simulink model "atrias_boom_nmSt_kinSw_v4"  (R2015a)
settings: Solver=ode23t  StartTime=0.0  StopTime=t_end  FixedStep=0.001  MaxStep=1e-3  RelTol=1e-3
InitFcn:
  | addpath('../common/')
  | colors
StartFcn:
  | tic
StopFcn:
  | %stopscript
values from neighbouring files (symbols this model uses):
  dt_a_dTrunk_boom = 5    [main_1_nmSt_kinSw.m]    (also in main_2_nmSt_kinSw_v2.m; main_3_nmSt_kinSw_v3.m; main_4_nmSt_kinSw_v4.m)
  dt_fade_boomCtrl = 2    [main_1_nmSt_kinSw.m]    (also in main_2_nmSt_kinSw_v2.m; main_3_nmSt_kinSw_v3.m; main_4_nmSt_kinSw_v4.m)
  initial_boom_yaw = 15*pi/180    (= 0.261799387799)    [main_2_nmSt_kinSw_v2.m]    (also in main_3_nmSt_kinSw_v3.m; main_4_nmSt_kinSw_v4.m)
  kd_boom_roll_Ctrl = 0    [main_1_nmSt_kinSw - Copy.m]    (also in main_1_nmSt_kinSw.m; main_2_nmSt_kinSw_v2.m; main_3_nmSt_kinSw_v3.m; main_4_nmSt_kinSw_v4.m)
  kd_boom_yaw_Ctrl = 0.1*kp_boom_yaw_Ctrl    (= 100000000)    [main_1_nmSt_kinSw - Copy.m]    (also in main_1_nmSt_kinSw.m = 1000000000; main_2_nmSt_kinSw_v2.m = 10000000; main_3_nmSt_kinSw_v3.m = 10000000; main_4_nmSt_kinSw_v4.m = 10000000)
  kd_motor = 0.90*2*sqrt(3.75*kp_motor)    [main_1_nmSt_kinSw - Copy.m]
  kinSw_alpha_start = 100*pi/180    (= 1.74532925199)    [main_1_nmSt_kinSw - Copy.m]    (also in main_1_nmSt_kinSw.m = 1.91986217719; main_2_nmSt_kinSw_v2.m = 1.83259571459; main_3_nmSt_kinSw_v3.m = 1.83259571459; main_4_nmSt_kinSw_v4.m = 1.83259571459)
  kinSw_alpha_tgt = 80*pi/180    (= 1.3962634016)    [main_1_nmSt_kinSw - Copy.m]    (also in main_1_nmSt_kinSw.m = 1.2217304764; main_2_nmSt_kinSw_v2.m = 1.2217304764; main_3_nmSt_kinSw_v3.m = 1.2217304764; main_4_nmSt_kinSw_v4.m = 1.2217304764)
  kinSw_t_start = 1.5    [main_1_nmSt_kinSw - Copy.m]    (also in main_1_nmSt_kinSw.m; main_2_nmSt_kinSw_v2.m = 0.5; main_3_nmSt_kinSw_v3.m = 0.5; main_4_nmSt_kinSw_v4.m = 0.5)
  kp_boom_roll_Ctrl = 0    [main_1_nmSt_kinSw - Copy.m]    (also in main_1_nmSt_kinSw.m; main_2_nmSt_kinSw_v2.m; main_3_nmSt_kinSw_v3.m; main_4_nmSt_kinSw_v4.m)
  kp_boom_yaw_Ctrl = 1e9    (= 1000000000)    [main_1_nmSt_kinSw - Copy.m]    (also in main_1_nmSt_kinSw.m = 10000000000; main_2_nmSt_kinSw_v2.m = 100000000; main_3_nmSt_kinSw_v3.m = 100000000; main_4_nmSt_kinSw_v4.m = 100000000)
  kp_motor = 3000    [main_1_nmSt_kinSw - Copy.m]
  max_back_bar_angle = 262.4*pi/180    (= 4.57974395723)    [main_1_nmSt_kinSw - Copy.m]
  max_front_bar_angle = 194.8*pi/180    (= 3.39990138288)    [main_1_nmSt_kinSw - Copy.m]
  min_back_bar_angle = 165.0*pi/180    (= 2.87979326579)    [main_1_nmSt_kinSw - Copy.m]
  min_front_bar_angle = 98.0*pi/180    (= 1.71042266695)    [main_1_nmSt_kinSw - Copy.m]
  poser_LLegAlp = (initial_l_leg_angle -pi/2)*180/pi    (= 105)    [main_2_nmSt_kinSw_v2.m]    (also in main_3_nmSt_kinSw_v3.m; main_4_nmSt_kinSw_v4.m)
  poser_LLegLen = initial_l_leg_length    (= 0.88)    [main_2_nmSt_kinSw_v2.m]    (also in main_3_nmSt_kinSw_v3.m; main_4_nmSt_kinSw_v4.m)
  poser_RLegAlp = (initial_r_leg_angle -pi/2)*180/pi    (= 75)    [main_2_nmSt_kinSw_v2.m]    (also in main_3_nmSt_kinSw_v3.m; main_4_nmSt_kinSw_v4.m)
  poser_RLegLen = initial_r_leg_length    (= 0.9)    [main_2_nmSt_kinSw_v2.m]    (also in main_3_nmSt_kinSw_v3.m; main_4_nmSt_kinSw_v4.m)
  tEnd_boomCtrl = t_end    (= 20)    [main_1_nmSt_kinSw - Copy.m]    (also in main_1_nmSt_kinSw.m = 3; main_2_nmSt_kinSw_v2.m = 7.5; main_3_nmSt_kinSw_v3.m = 7.5; main_4_nmSt_kinSw_v4.m = 7.5)
  tStart_boomCtrl = 1    [main_1_nmSt_kinSw - Copy.m]    (also in main_1_nmSt_kinSw.m = 0; main_2_nmSt_kinSw_v2.m = 0.5; main_3_nmSt_kinSw_v3.m = 0.5; main_4_nmSt_kinSw_v4.m = 0.5)
  tune_kinSw_alpha_start = kinSw_alpha_start*180/pi    (= 105)    [main_2_nmSt_kinSw_v2.m]    (also in main_3_nmSt_kinSw_v3.m; main_4_nmSt_kinSw_v4.m)
  tune_kinSw_alpha_tgt = kinSw_alpha_tgt*180/pi    (= 70)    [main_2_nmSt_kinSw_v2.m]    (also in main_3_nmSt_kinSw_v3.m; main_4_nmSt_kinSw_v4.m)
  tune_kinSw_gClr_tgt = kinSw_gClr    (= 0.15)    [main_4_nmSt_kinSw_v4.m]
  tune_kinSw_gH_tgt = kinSw_gH_tgt    (= -0.01)    [main_4_nmSt_kinSw_v4.m]
  tune_M1_G = St_FGain_VAS*FmaxVAS    [main_2_nmSt_kinSw_v2.m]    (also in main_3_nmSt_kinSw_v3.m; main_4_nmSt_kinSw_v4.m)
  tune_M3_0 = CtrlPar_theta0*180/pi    [main_2_nmSt_kinSw_v2.m]    (also in main_3_nmSt_kinSw_v3.m; main_4_nmSt_kinSw_v4.m)
  tune_M3_D = St_GainDTh_HFL    [main_2_nmSt_kinSw_v2.m]    (also in main_3_nmSt_kinSw_v3.m; main_4_nmSt_kinSw_v4.m)
  tune_M3_P = St_GainTh_HFL    [main_2_nmSt_kinSw_v2.m]    (also in main_3_nmSt_kinSw_v3.m; main_4_nmSt_kinSw_v4.m)
  tune_M4_G = 1    [main_3_nmSt_kinSw_v3.m]    (also in main_4_nmSt_kinSw_v4.m)
  v_dTrunk_boom = 1.3    [main_1_nmSt_kinSw.m]    (also in main_2_nmSt_kinSw_v2.m; main_3_nmSt_kinSw_v3.m; main_4_nmSt_kinSw_v4.m)
undefined symbols (not defined in the file or in its folder): A1_notch_f1, A2_notch_f1, A_lpf_dtau, A_lpf_velocity, ankle_stiffness, B1_lpf_dtau, B1_lpf_velocity, B1_notch_f1, B2_lpf_dtau, B2_lpf_velocity, B2_notch_f1, b_hmotor, b_leg_spring, b_rotor, base_color_d, boom_color_d, boom_mount_to_center_diagonal, breakaway_friction, c_jointstop, contactThr, coulomb_friction, d_com, delta_phi_max, delta_phi_max_buffer, delta_phi_max_dropoff, delta_phi_min, fblink_color_d, floor_color_d, FmaxBFSH, FmaxGLU, FmaxHAM, FmaxHFL, FmaxRF, FmaxVAS, foot_color_d, FPCtrlPar, friction_linear_zone, g, gain_nodes_sea_torque, HIP_MTR_MAX_CONT_TORQUE, HIP_MTR_MAX_TORQUE, hshaft_color_d, initial_boom_pitch, initial_boom_roll, initial_hip_roll, initial_winch_angle, j_motor, k_gn, k_gt, k_leg_spring, K_notch_f1, k_phi, k_sea, Kb_leg, kd_lateral, kd_shin_max, kd_shin_min, kd_splay_max, kd_splay_min, kd_thigh_max ... (+186)
libraries: sm_lib x210, nesl_utility x140, simulink x65, simulink_extras x32, fl_lib x16, mblibv1 x2, commnoisgen2 x1
(part 17 of 17)

== system atrias_boom_nmSt_kinSw_v4/Control/Behavior Control/Virtual Neuromuscular Control/Torque Distribution/mech limit avoidance1/PD Joint Limit1/R scale desired torque1 ==
  note: NOTE: min_splay_angle does not equal delta_phi_min
  phi_thigh [rad] : Inport
  phi_shin [rad] : Inport  Port=2
  k : Inport  Port=3
  Constant : Constant
  Constant1 : Constant  Value=delta_phi_max - delta_phi_max_buffer
  Constant10 : Constant  Value=phi_thigh_max_buffer
  Constant11 : Constant  Value=phi_shin_min_buffer
  Constant12 : Constant  Value=phi_shin_max_buffer
  Constant13 : Constant
  Constant2 : Constant  Value=phi_thigh_max - phi_thigh_max_buffer
  Constant3 : Constant  Value=min_splay_angle
  Constant4 : Constant  Value=phi_thigh_min + phi_thigh_min_buffer
  Constant5 : Constant  Value=phi_shin_max - phi_shin_max_buffer
  Constant6 : Constant  Value=phi_shin_min + phi_shin_min_buffer
  Constant7 : Constant  Value=min_splay_angle - delta_phi_min
  Constant8 : Constant  Value=delta_phi_max_buffer
  Constant9 : Constant  Value=phi_thigh_min_buffer
  Demux : Demux  Outputs=2
  Divide{,1..5} (6 alike) : Product  Inputs=/*
  Gain : Gain  Gain=-1
  Gain1 : Gain  Gain=-1
  Gain2 : Gain  Gain=-1
  L scale hip/knee : Scope  NumInputPorts=4
      settings: ShowLegends=on  TimeRange=2.5  YMin=-100~-5e+07~-1e+07~-5  YMax=100~1e+07~5e+07~5  SaveName=ScopeData5
  Mux{,3,7..8} (4 alike) : Mux  Inputs=2
  Sum : Sum  Inputs=|+-
  Sum1 : Sum  Inputs=-+|
  Sum2 : Sum  Inputs=+-
  Sum{3..8} (6 alike) : Sum  Inputs=+-|
  [0,1]{,1..6} (7 alike) : Saturate  UpperLimit=1  LowerLimit=0
  max : MinMax  Function=max  Inputs=4
  max1 : MinMax  Function=max  Inputs=4
  to hip_knee : MATLAB Function  TreatAsAtomicUnit=on
  scale_hip : Outport
  scale_knee : Outport  Port=2
  wires:
  "[0,1]6"/1 -> Demux/1
  Mux3/1 -> L scale hip/knee/4
  Demux/2 -> Sum1/1
  Demux/1 -> Sum/2
  to hip_knee/1(scale_hip_knee) -> "[0,1]6"/1
  k/1 -> to hip_knee/3(k)
  max1/1 -> to hip_knee/2(scale_front)
  max/1 -> to hip_knee/1(scale_back)
  Sum1/1 -> scale_knee/1, Mux3/2
  [min_thigh_scale] -> max1/3
  [max_thigh_scale] -> max1/4
  [max_splay_scale] -> max/4, max1/2
  [min_splay_scale] -> max/3, max1/1
  [max_shin_scale] -> max/2
  [min_shin_scale] -> max/1
  Constant13/1 -> Sum1/2
  Gain2/1 -> Divide5/2
  Constant12/1 -> Divide5/1
  Sum7/1 -> Gain2/1
  "[0,1]5"/1 -> [max_shin_scale]
  Divide5/1 -> "[0,1]5"/1
  Constant11/1 -> Divide4/1
  Sum8/1 -> Divide4/2
  "[0,1]4"/1 -> [min_shin_scale]
  Divide4/1 -> "[0,1]4"/1
  Constant10/1 -> Divide3/1
  Sum5/1 -> Gain1/1
  Gain1/1 -> Divide3/2
  "[0,1]3"/1 -> [max_thigh_scale]
  Divide3/1 -> "[0,1]3"/1
  Constant9/1 -> Divide2/1
  Sum6/1 -> Divide2/2
  "[0,1]2"/1 -> [min_thigh_scale]
  Divide2/1 -> "[0,1]2"/1
  Gain/1 -> Divide1/2
  Constant8/1 -> Divide1/1
  Sum3/1 -> Gain/1
  "[0,1]1"/1 -> [max_splay_scale]
  Divide1/1 -> "[0,1]1"/1
  "[0,1]"/1 -> [min_splay_scale]
  Divide/1 -> "[0,1]"/1
  Sum4/1 -> Divide/2
  Constant7/1 -> Divide/1
  Constant/1 -> Sum/1
  Sum/1 -> scale_hip/1, Mux3/1
  [max_splay_scale] -> Mux7/2  "max_splay_trq"
  [min_splay_scale] -> Mux7/1  "min_splay_trq"
  Mux7/1 -> L scale hip/knee/3
  Mux8/1 -> L scale hip/knee/2
  [max_shin_scale] -> Mux8/2  "max_shin_trq"
  [min_shin_scale] -> Mux8/1  "min_shin_trq"
  Mux/1 -> L scale hip/knee/1
  [max_thigh_scale] -> Mux/2  "max_thigh_trq"
  [min_thigh_scale] -> Mux/1  "min_thigh_trq"
  Constant5/1 -> Sum7/1
  [shin] -> Sum7/2
  Constant6/1 -> Sum8/1
  [shin] -> Sum8/2
  Constant2/1 -> Sum5/1
  [thigh] -> Sum5/2
  Constant4/1 -> Sum6/1
  [thigh] -> Sum6/2
  Constant1/1 -> Sum3/1
  [splay] -> Sum3/2
  Constant3/1 -> Sum4/1
  [splay] -> Sum4/2
  Sum2/1 -> [splay]  "splay angle"
  phi_thigh [rad]/1 -> Sum2/2, [thigh]
  phi_shin [rad]/1 -> Sum2/1, [shin]

== matlab function atrias_boom_nmSt_kinSw_v4/Control/Behavior Control/Virtual Neuromuscular Control/Torque Distribution/mech limit avoidance1/PD Joint Limit1/R scale desired torque/to hip_knee ==
  data: scale_back input; scale_hip_knee output; scale_front input; k input
function scale_hip_knee = fcn(scale_back,scale_front,k)

J_inv_trans = [1,1;
               -((k+1)/(2*k)),-((k-1)/(2*k))];
           
scale_hip_knee = J_inv_trans*[scale_back;scale_front];

== matlab function atrias_boom_nmSt_kinSw_v4/Control/Behavior Control/Virtual Neuromuscular Control/Torque Distribution/map_tau_R ==
  settings: updateMethod=DISCRETE  sampleTime=sample_time
  data: tauH_des input; tauB output; tauK_des input; tauF output; k input; Jinv_trans output
function [tauB,tauF, Jinv_trans] = map_virtual_torques(tauH_des,tauK_des,k)
%% FOR REFERENCE: 
%   [dphi_hip; dphi_knee] = J * [dq_back; dq_front];
%   
%   [dq_back; dq_front] = J^(-1) * [dphi_hip; dphi_knee];
%
%   [tauB; tauF] = Jt * [tauH, tauK]
%   
%   [tauH, tauK] = Jt^(-1) * [tauB; tauF]
%
%   J = [(1-k)/2    (1+k)/2 ]   where   k = l_s*sin((q_back-q_front)/2) /
%       [-k         k       ]               l_v*cos(phi_knee/2)
%
% 

%% Construct jacobian, then map virtual torques to actuator torques
j11 = (1-k)/2;
j12 = (1+k)/2;
j21 = -k;
j22 = k;

J = [j11, j12; j21, j22]; 
Jinv_trans = inv(J)';

tau_q = J'*[tauH_des; tauK_des];

tauB = tau_q(1);
tauF = tau_q(2);

end

== matlab function atrias_boom_nmSt_kinSw_v4/Control/Behavior Control/Virtual Neuromuscular Control/Torque Distribution/mech limit avoidance1/PD Joint Limit1/R scale desired torque1/to hip_knee ==
  data: scale_back input; scale_hip_knee output; scale_front input; k input
function scale_hip_knee = fcn(scale_back,scale_front,k)

J_inv_trans = [1,1;
               -((k+1)/(2*k)),-((k-1)/(2*k))];
           
scale_hip_knee = J_inv_trans*[scale_back;scale_front];

== matlab function atrias_boom_nmSt_kinSw_v4/Control/Behavior Control/Virtual Neuromuscular Control/Torque Distribution/map_tau_L ==
  settings: updateMethod=DISCRETE  sampleTime=sample_time
  data: tauH_des input; tauB output; tauK_des input; tauF output; k input; Jinv_trans output
function [tauB,tauF, Jinv_trans] = map_virtual_torques(tauH_des,tauK_des,k)
%% FOR REFERENCE: 
%   [dphi_hip; dphi_knee] = J * [dq_back; dq_front];
%   
%   [dq_back; dq_front] = J^(-1) * [dphi_hip; dphi_knee];
%
%   [tauB; tauF] = Jt * [tauH, tauK]
%   
%   [tauH, tauK] = Jt^(-1) * [tauB; tauF]
%
%   J = [(1-k)/2    (1+k)/2 ]   where   k = l_s*sin((q_back-q_front)/2) /
%       [-k         k       ]               l_v*cos(phi_knee/2)
%
% 

%% Construct jacobian, then map virtual torques to actuator torques
j11 = (1-k)/2;
j12 = (1+k)/2;
j21 = -k;
j22 = k;

J = [j11, j12; j21, j22]; 
Jinv_trans = inv(J)';

tau_q = J'*[tauH_des; tauK_des];

tauB = tau_q(1);
tauF = tau_q(2);

end

== matlab function atrias_boom_nmSt_kinSw_v4/Control/Behavior Control/Virtual Neuromuscular Control/Torque Distribution/mech limit avoidance1/PD Joint Limit1/to hip_knee ==
  data: Rtau_back input; tau_pd_hip_knee output; Rtau_front input; Ltau_back input; Ltau_front input; kR input; kL input
function tau_pd_hip_knee = fcn(Rtau_back,Rtau_front,Ltau_back,Ltau_front,kR,kL)

J_inv_trans = [1,1,0,0;
               -((kR+1)/(2*kR)),-((kR-1)/(2*kR)),0,0;
               0,0,1,1;
               0,0,-((kL+1)/(2*kL)),-((kL-1)/(2*kL))];
           
tau_pd_hip_knee = J_inv_trans*[Rtau_back;
                               Rtau_front;
                               Ltau_back;
                               Ltau_front];

== matlab function atrias_boom_nmSt_kinSw_v4/Control/Behavior Control/Lateral Motor Control/Lateral Control1 ==
  data: tau_r output size=1; qLateralR input; dqLateralR input; qLateralL input; dqLateralL input; F_leg_R input; F_leg_L input; lateral_transition_force parameter; lateral_target_angle_right parameter; m_leg_motor parameter; m_leg parameter; g parameter; lateral_offset parameter; tau_l output size=1; kp_lateral parameter; kd_lateral parameter; minimum_lateral_angle parameter; maximum_lateral_angle parameter; HIP_MTR_MAX_CONT_TORQUE parameter
function [tau_r, tau_l] = LateralBoomControl(...
    qLateralR, dqLateralR, qLateralL, dqLateralL, F_leg_R, F_leg_L,...
    lateral_transition_force, lateral_target_angle_right,...
    m_leg_motor, m_leg, g, lateral_offset,...
    kp_lateral, kd_lateral, minimum_lateral_angle, maximum_lateral_angle, HIP_MTR_MAX_CONT_TORQUE)
    
    % Only add gravity compensation to PD when suspended from winch (approximately static)
    gravity_compensation = 0;
    
    % Inertia for feedforward accelerations
    motor_inertia = (m_leg_motor+m_leg)*lateral_offset^2;
    
    % Right Leg
    right_target = [lateral_target_angle_right, 0, 0];
    desired = [saturate(right_target(1),minimum_lateral_angle,maximum_lateral_angle), right_target(2)];
    measured = [qLateralR, dqLateralR];
    tau_r = [kp_lateral, kd_lateral] * (desired-measured)' + gravity_compensation + motor_inertia*right_target(3);
    tau_r = max(min(HIP_MTR_MAX_CONT_TORQUE, tau_r),-HIP_MTR_MAX_CONT_TORQUE);
    
    if (F_leg_R >= lateral_transition_force)
        tau_r = -lateral_offset*(F_leg_R-(m_leg_motor+m_leg)*g);
    end
    
    % Left Leg
    left_target = [lateral_target_angle_right, 0, 0];
    desired = [saturate(left_target(1),minimum_lateral_angle,maximum_lateral_angle), left_target(2)];
    measured = [qLateralL, dqLateralL];
    tau_l = [kp_lateral, kd_lateral] * (desired-measured)' + gravity_compensation + motor_inertia*left_target(3);
    tau_l = max(min(HIP_MTR_MAX_CONT_TORQUE, tau_l),-HIP_MTR_MAX_CONT_TORQUE);
    
    if (F_leg_L >= lateral_transition_force)
        tau_l = -lateral_offset*(F_leg_L-(m_leg_motor+m_leg)*g);
    end
end

function [desired_saturated] = saturate(desired, minimum_lateral_angle, maximum_lateral_angle)
    desired_saturated = desired;
    if desired(1) < minimum_lateral_angle
        desired_saturated = [minimum_lateral_angle, 0];
    elseif desired(1) > maximum_lateral_angle
        desired_saturated = [maximum_lateral_angle, 0];    
    end
end

== matlab function atrias_boom_nmSt_kinSw_v4/Control/Behavior Control/kinematic swing leg controller/Avoid Hitting Mechanical Limits ==
  data: back_cmd output double; front_cmd output double; dback_cmd output double; dfront_cmd output double; ddback_cmd output double; ddfront_cmd output double; back_desired input; dback_desired input; ddback_desired input; front_desired input; dfront_desired input; ddfront_desired input; min_front_bar_angle input; max_front_bar_angle input; min_back_bar_angle input; max_back_bar_angle input
%% Avoid joint limits by ensuring we don't command velocities/accelerations that would push us into them when we are close to them.
function [back_cmd, front_cmd, dback_cmd, dfront_cmd, ddback_cmd, ddfront_cmd] ...
    = AvoidFourbarLimits(back_desired,dback_desired, ddback_desired, ...
          front_desired, dfront_desired, ddfront_desired, ...
          min_front_bar_angle, max_front_bar_angle, min_back_bar_angle, max_back_bar_angle)
    [back_cmd, front_cmd, dback_cmd, dfront_cmd, ddback_cmd, ddfront_cmd] = AvoidFourbarLimits(back_desired,dback_desired, ddback_desired, front_desired, dfront_desired, ddfront_desired, min_front_bar_angle, max_front_bar_angle, min_back_bar_angle, max_back_bar_angle);
end

== matlab function atrias_boom_nmSt_kinSw_v4/Control/Behavior Control/kinematic swing leg controller/Generate Parabolic Trajectories ==
  data: legLen_ref output size=3; flight input; hipHeight input; gH0 input; gclr_tgt input; gH_star input; alpha_start input; alpha_star input; alpha input
%% Parabolic trajectory generation for leg angle and length
% est_duration: estimated flight time
% time_remaining: time until estimated touchdown
% legAlp0: legAlp at takeoff
%   legAlp is the angle of attack
% legLen0: legLen at takeoff
% legAlp_star: desired legAlp
% legLen_star: desired legLen
% legLen_min: min legLen for ground clearance
% min_f_duration: minimum trajectory time

function legLen_ref   =  ...
          GenerateReferenceLegLength(flight, hipHeight,...
                    gH0, gclr_tgt, gH_star,   ...
                    alpha_start, alpha_star, alpha)

if ~flight || alpha == 0
    legLen_ref = [0.9;0;0];
    return;
end

    
  % split duration into thirds.  First segment: parabola from legLen0 to
  % legLen_min.  Second and third segments, cos to landing.
  alpha_d   = abs(alpha_star-alpha_start);
  alpha_r   = max(abs(alpha_star-alpha), 0);
  da3 = alpha_d / 3;
  if alpha_r > 2*da3;
    gClr_star_a = gclr_tgt + (gH0-gclr_tgt)*((alpha_r-2*da3)/da3)^2;
    dgClr_star_a = -(gH0-gclr_tgt)*2*(alpha_r-2*da3)/da3/da3;
    ddgClr_star_a = (gH0-gclr_tgt)*2/da3^2;
  else
    gClr_star_a = gH_star + (gclr_tgt-gH_star)/2*(1-cos(alpha_r/(2*da3)*pi));
    dgClr_star_a = -(gclr_tgt-gH_star)/2*sin(alpha_r/(2*da3)*pi)*pi/(2*da3);
    ddgClr_star_a = (gclr_tgt-gH_star)/2*cos(alpha_r/(2*da3)*pi)*(pi/(2*da3))^2;
  end
  
  legLenV_star      = hipHeight - gClr_star_a;
  legLen_star_a   	= legLenV_star/sin(alpha);
  dlegLen_star_a    = -dgClr_star_a/sin(alpha);
  ddlegLen_star_a   = -ddgClr_star_a/sin(alpha);
  
  % track a sinusoidal z of amplitude max_retract, finishing a half-cycle by t_end
  legLen_ref = [legLen_star_a; dlegLen_star_a; ddlegLen_star_a];

== matlab function atrias_boom_nmSt_kinSw_v4/Control/Behavior Control/kinematic swing leg controller/Virtual Leg to Four Bar ==
  data: l_leg input; dl_leg input; ddl_leg input; phi input; dphi input; ddphi input; back output; dback output; ddback output; front output; dfront output; ddfront output
function [back, dback, ddback, front, dfront, ddfront] = VirtualLegToFourBar(l_leg, dl_leg, ddl_leg, phi, dphi, ddphi)
    [back, dback, ddback, front, dfront, ddfront] = VirtualLegToFourBar(l_leg, dl_leg, ddl_leg, phi, dphi, ddphi);
end
